simulink model "raddi_est_2013b"  (R2013b)
settings: Solver=ode45  StartTime=0.0  StopTime=inf  RelTol=1e-3
settings Model: Creator=igeorgie  LastModifiedBy=igeorgie
settings DebuggingCC: FrameProcessingCompatibilityMsg=error
settings GRTTargetCC: CodeReplacementLibrary=C89/C90 (ANSI)

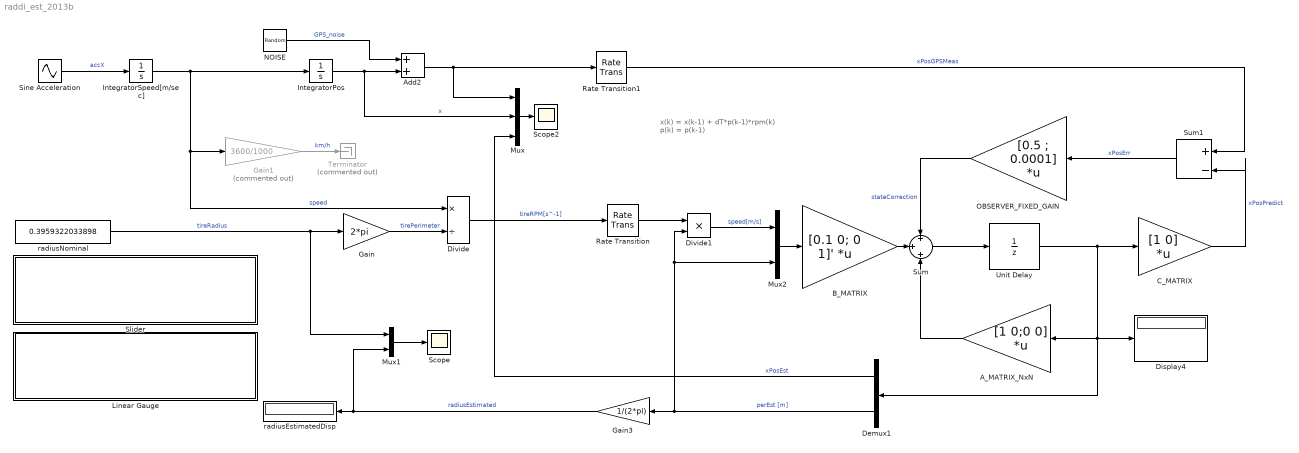
== system raddi_est_2013b ==
  note: x(k) = x(k-1) + dT*p(k-1)*rpm(k)
      | p(k) = p(k-1)
  A_MATRIX_NxN : Gain  Gain=[1 0;0 0]  Multiplication=Matrix(K*u)
  Add2 : Sum
  B_MATRIX : Gain  Gain=[0.1 0; 0 1]'  Multiplication=Matrix(K*u)
  C_MATRIX : Gain  Gain=[1 0]  Multiplication=Matrix(K*u)
  Demux1 : Demux  Outputs=2
  Display4 : Display
  Divide : Product  Inputs=*/
  Divide1 : Product  Inputs=**
  Gain : Gain  Gain=2*pi
  Gain1 : Gain  Commented=on  Gain=3600/1000
  Gain3 : Gain  Gain=1/(2*pi)
  IntegratorPos : Integrator
  IntegratorSpeed[m/sec] : Integrator
  Linear Gauge : Subsystem  Description=Replaced Block  mask(Replaced Block){}
      mask help: This block has been replaced with an empty subsystem because it used functionality that is unavailable in Simulink R2013b.
      mask Display: fprintf('Replaced: %s\n','Dashboard Widget')
  Mux : Mux  Inputs=3
  Mux1 : Mux  Inputs=2
  Mux2 : Mux  Inputs=2
  NOISE : RandomNumber  Variance=2000  SampleTime=0.1
  OBSERVER_FIXED_GAIN : Gain  Gain=[0.5 ; 0.0001]  Multiplication=Matrix(K*u)
  Rate Transition : RateTransition  OutPortSampleTime=0.1
  Rate Transition1 : RateTransition  OutPortSampleTime=0.1
  Scope : Scope
      settings: TimeRange=50000  MaxDataPoints=5000  SaveToWorkspace=off  YMin=0  YMax=1  SampleTime=-1
  Scope2 : Scope
      settings: TimeRange=auto  LimitDataPoints=on  MaxDataPoints=500000  SaveToWorkspace=off  SaveName=ScopeData2  YMin=3298872.55351  YMax=4378100.40264  SampleTime=-1
  Sine Acceleration : Sin  Amplitude=0.03  Frequency=2*pi*(1/3600)
  Slider : Subsystem  Description=Replaced Block  mask(Replaced Block){}
      mask help: This block has been replaced with an empty subsystem because it used functionality that is unavailable in Simulink R2013b.
      mask Display: fprintf('Replaced: %s\n','Dashboard Widget')
  Sum : Sum  Inputs=+|+|+
  Sum1 : Sum  Inputs=+-|
  Terminator : Terminator  Commented=on
  Unit Delay : UnitDelay  InitialCondition=[1000 2]  SampleTime=-1
  radiusEstimatedDisp : Display
  radiusNominal : Constant  Value=0.3959322033898
  wires:
  Sine Acceleration/1 -> IntegratorSpeed[m/sec]/1  "accX"
  IntegratorPos/1 -> Mux/2, Add2/2  "x"
  IntegratorSpeed[m/sec]/1 -> IntegratorPos/1, Divide/1, Gain1/1  "speed"
  Gain/1 -> Divide/2  "tirePerimeter"
  radiusNominal/1 -> Gain/1, Mux1/1  "tireRadius"
  Divide/1 -> Rate Transition/1  "tireRPM[s^-1]"
  Rate Transition/1 -> Divide1/1
  A_MATRIX_NxN/1 -> Sum/3
  Sum/1 -> Unit Delay/1
  Unit Delay/1 -> Demux1/1, Display4/1, A_MATRIX_NxN/1, C_MATRIX/1
  C_MATRIX/1 -> Sum1/2  "xPosPredict"
  Sum1/1 -> OBSERVER_FIXED_GAIN/1  "xPosErr"
  OBSERVER_FIXED_GAIN/1 -> Sum/1  "stateCorrection"
  Mux/1 -> Scope2/1
  Demux1/1 -> Mux/3  "xPosEst"
  Demux1/2 -> Mux2/2, Divide1/2, Gain3/1  "perEst [m]"
  Rate Transition1/1 -> Sum1/1  "xPosGPSMeas"
  B_MATRIX/1 -> Sum/2
  Divide1/1 -> Mux2/1  "speed[m/s]"
  Mux2/1 -> B_MATRIX/1
  Add2/1 -> Mux/1, Rate Transition1/1
  NOISE/1 -> Add2/1  "GPS_noise"
  Gain3/1 -> Mux1/2, radiusEstimatedDisp/1  "radiusEstimated"
  Mux1/1 -> Scope/1
  Gain1/1 -> Terminator/1  "km/h"

== system raddi_est_2013b/Linear Gauge ==

== system raddi_est_2013b/Slider ==
